simulink library "ESSLibrary"  (R2020a)
settings: Solver=VariableStepAuto  StartTime=0.0  StopTime=10.0  RelTol=1e-3
libraries: $bdroot x82, powerlib_meascontrol x10, simulink x7
(part 1 of 7)
settings Model: Creator=ASHUTOSHKUMARTIWARI  LastModifiedBy=soumyakantapanda

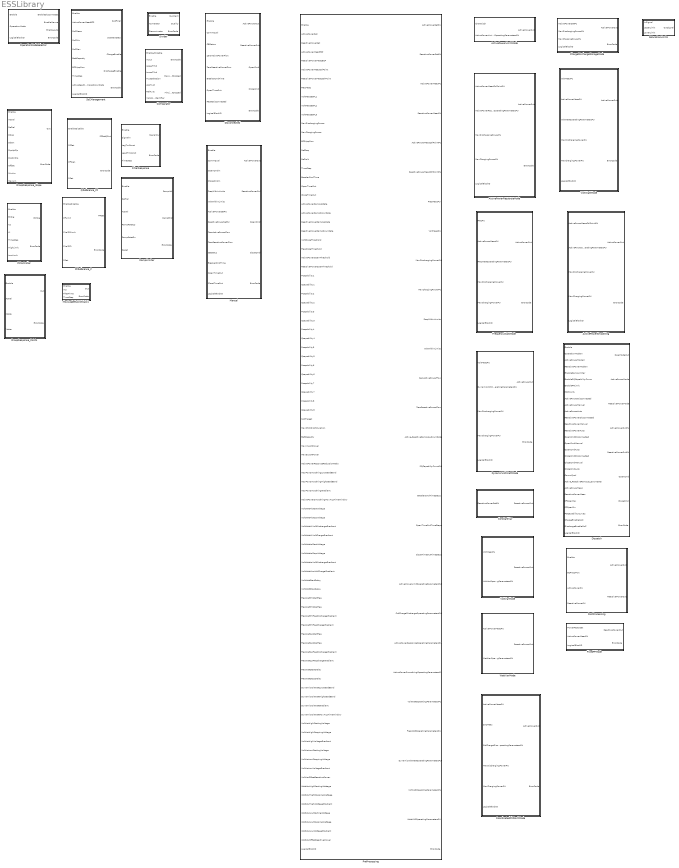
== system ESSLibrary ==
  ActivePowerLimitMode : Subsystem  RTWFcnName=ActivePowerLimitMode
      settings: RTWFcnNameOpts=User specified  RTWFileNameOpts=Use function name
  ActivePowerResponseMode : Subsystem  TreatAsAtomicUnit=on
  ActivePowerSmoothing : Subsystem
  ChargeDischargeStorageMode : Subsystem
  Comparator : Subsystem
  ConstantVar : Subsystem
  CoordinatedChDischMode : Subsystem
  Disconnected : Subsystem  TreatAsAtomicUnit=on  RTWFcnName=Disconnected
      settings: RTWFcnNameOpts=User specified  RTWFileNameOpts=Use function name
  Dispatch : Subsystem
  Divider : Subsystem  TreatAsAtomicUnit=on  RTWFcnName=Divider
      settings: RTWFcnNameOpts=User specified  RTWFileNameOpts=Use function name
  DroopResponse_Points : Subsystem  TreatAsAtomicUnit=on
  DroopResponse_Slope : Subsystem  TreatAsAtomicUnit=on
  DynamicVoltWattMode : Subsystem
  FilterResponse : Subsystem
  FixedPFMode : Subsystem
  FrequencyWattMode : Subsystem  TreatAsAtomicUnit=on
  Manual : Subsystem  TreatAsAtomicUnit=on  RTWFcnName=Manual
      settings: RTWFcnNameOpts=User specified  RTWFileNameOpts=Use function name
  MovAvgDeltaVoltCalc1 : Subsystem
  OperationModeSelector : Subsystem  TreatAsAtomicUnit=on  RTWFcnName=OperationModeSelector
      settings: RTWFcnNameOpts=User specified  RTWFileNameOpts=Use function name
  PFReference_P : Subsystem  TreatAsAtomicUnit=on
  PIController : Subsystem  TreatAsAtomicUnit=on
  PostProcessing : Subsystem
  PreProcessing : Subsystem  TreatAsAtomicUnit=on  RTWFcnName=PreProcessing
      settings: RTWFcnNameOpts=User specified  RTWFileNameOpts=Use function name
  QReference_PF : Subsystem  TreatAsAtomicUnit=on
  RampLimiter : MATLAB Function  TreatAsAtomicUnit=on
  SaturationLimits : Subsystem
  SoCManagement : Subsystem  TreatAsAtomicUnit=on  RTWFcnName=SoCManagement
      settings: RTWFcnNameOpts=User specified  RTWFileNameOpts=Use function name
  VoltVarMode : Subsystem
  VoltWattMode : Subsystem
  WattVarMode : Subsystem

== system ESSLibrary/ActivePowerLimitMode ==
  ChOrDisch : Inport  OutDataTypeStr=double
  ActivePowerLimitOperatingParametersPU : Inport  Port=2  OutDataTypeStr=Bus: ActivePowerLimitOperatingParametersPU
  Action Port : ActionPort
  Bus Selector1 : BusSelector  OutputSignals=MaxDischargingPowerPU,MaxChargingPowerPU
  Switch : Switch  Criteria=u2 > Threshold
  ActivePowerOut : Outport
  wires:
  ChOrDisch/1 -> Switch/2
  Switch/1 -> ActivePowerOut/1
  ActivePowerLimitOperatingParametersPU/1 -> Bus Selector1/1
  Bus Selector1/1 -> Switch/1  "<MaxDischargingPowerPU>"
  Bus Selector1/2 -> Switch/3  "<MaxChargingPowerPU>"

== system ESSLibrary/ActivePowerResponseMode ==
  ActivePowerMeasCtrlPointPU : Inport  OutDataTypeStr=double
  ActivePowerResponseOperatingParametersPU : Inport  Port=2  OutDataTypeStr=Bus: ActivePowerResponseOperatingParametersPU
  MaxDischargingPowerPU : Inport  Port=3  OutDataTypeStr=double
  MaxChargingPowerPU : Inport  Port=4  OutDataTypeStr=double
  LogicalBlockID : Inport  Port=5  OutDataTypeStr=int64
  Action Port : ActionPort
  ActivePowerMeasCtrlPointPU1 : InportShadow  OutDataTypeStr=double
  Bus Selector6 : BusSelector  OutputSignals=MaxExportPowerPU,MaxImportPowerPU,ReductionRatio
  Comparator : $bdroot/ChargeDischargeStorageMode/Comparator  SystemSampleTime=-1  Latency=0  AutoFrameSizeCalculation=off
  Constant10 : Constant  Value=0  OutDataTypeStr=int64
  Constant11 : Constant  Value=0  OutDataTypeStr=int64
  Constant2 : Constant  Value=2  OutDataTypeStr=int32
  Constant3 : Constant  Value=0  OutDataTypeStr=int8
  Constant5 : Constant  Value=0  OutDataTypeStr=int8
  Constant6 : Constant  OutDataTypeStr=boolean
  Divide1 : Product  Inputs=**
  Divide2 : Product  Inputs=**
  Equal2 : RelationalOperator  Operator=>  OutDataTypeStr=boolean  RndMeth=Simplest
  Gain1 : Gain  Gain=1000000
  Less Than : RelationalOperator  OutDataTypeStr=boolean  RndMeth=Simplest
  Less Than1 : RelationalOperator  Operator=<=  OutDataTypeStr=boolean  RndMeth=Simplest
  MaxChargingPowerPU1 : InportShadow  Port=4  OutDataTypeStr=double
  MaxDischargingPowerPU1 : InportShadow  Port=3  OutDataTypeStr=double
  SaturationLimits : $bdroot/SaturationLimits  SystemSampleTime=-1  Latency=0  AutoFrameSizeCalculation=off
  Sum : Sum  Inputs=|+-
  Sum1 : Sum  Inputs=|-+
  Sum2 : Sum  OutDataTypeStr=int64
  Switch : Switch  Criteria=u2 > Threshold  OutDataTypeStr=double
  Switch1 : Switch  Criteria=u2 > Threshold  OutDataTypeStr=double
  Switch4 : Switch  Criteria=u2 > Threshold
  Terminator : Terminator
  Terminator1 : Terminator
  VariableIdentifier : Constant  OutDataTypeStr=int64
  Zero : Constant  Value=0.0  OutDataTypeStr=double
  ActivePowerOut : Outport
  ErrorCode : Outport  Port=2  OutDataTypeStr=int64
  wires:
  [ReductionRatio] -> Divide1/2
  Divide1/1 -> Switch/1
  Less Than/1 -> Switch/2
  Sum/1 -> Divide1/1
  ActivePowerResponseOperatingParametersPU/1 -> Bus Selector6/1
  Bus Selector6/1 -> [MaxExportPowerPU]  "<MaxExportPowerPU>"
  Bus Selector6/2 -> [MaxImportPowerPU]  "<MaxImportPowerPU>"
  ActivePowerMeasCtrlPointPU/1 -> Sum/1, Less Than/1
  [MaxExportPowerPU] -> Less Than/2, Sum/2
  Bus Selector6/3 -> [ReductionRatio]  "<ReductionRatio>"
  [MaxImportPowerPU] -> Sum1/2, Less Than1/2
  ActivePowerMeasCtrlPointPU1/1 -> Sum1/1, Less Than1/1
  Less Than1/1 -> Switch1/2
  Switch1/1 -> Switch/3
  Sum1/1 -> Divide2/1
  [ReductionRatio] -> Divide2/2
  Divide2/1 -> Switch1/1
  Zero/1 -> Switch1/3
  Switch/1 -> SaturationLimits/1, Comparator/2
  SaturationLimits/1 -> ActivePowerOut/1
  MaxDischargingPowerPU/1 -> SaturationLimits/2
  MaxChargingPowerPU/1 -> SaturationLimits/3
  Constant10/1 -> Equal2/2
  Sum2/1 -> Switch4/1
  Constant3/1 -> Comparator/6
  Gain1/1 -> Sum2/2
  Equal2/1 -> Switch4/2
  Comparator/1 -> Equal2/1, Sum2/1
  Switch4/1 -> ErrorCode/1
  Constant6/1 -> Comparator/1
  Comparator/2 -> Terminator/1
  Constant11/1 -> Switch4/3
  VariableIdentifier/1 -> Comparator/8
  LogicalBlockID/1 -> Gain1/1
  Constant5/1 -> Comparator/7
  Constant2/1 -> Comparator/5
  Comparator/3 -> Terminator1/1
  MaxDischargingPowerPU1/1 -> Comparator/3
  MaxChargingPowerPU1/1 -> Comparator/4

== system ESSLibrary/ActivePowerSmoothing ==
  ActivePowerMeasCtrlPointPU : Inport
  ActivePowerSmoothingOperatingParametersPU : Inport  Port=2  OutDataTypeStr=Bus: ActivePowerSmoothingParametersPU
  MaxDischargingPowerPU : Inport  Port=3  OutDataTypeStr=double
  MaxChargingPowerPU : Inport  Port=4  OutDataTypeStr=double
  LogicalBlockID : Inport  Port=5  OutDataTypeStr=int64
  Action Port : ActionPort
  ActivePowerMeasCtrlPointPU1 : InportShadow
  Bus Selector2 : BusSelector  OutputSignals=ActivePowerSmoothingLowDeadBandPU,ActivePowerSmoothingHighDeadBandPU,ActivePowerSmoothingGradientPU,ActivePowerSmoothingMovAvgTimeWindow,TimeStep
  Comparator : $bdroot/ChargeDischargeStorageMode/Comparator  SystemSampleTime=-1  Latency=0  AutoFrameSizeCalculation=off
  Constant1 : Constant  Value=0.0  OutDataTypeStr=double  SampleTime=-1
  Constant10 : Constant  Value=0  OutDataTypeStr=int64
  Constant11 : Constant  Value=0  OutDataTypeStr=int64
  Constant2 : Constant  Value=0.0  OutDataTypeStr=double  SampleTime=-1
  Constant3 : Constant  OutDataTypeStr=boolean
  Constant4 : Constant  Value=2  OutDataTypeStr=int32
  Constant5 : Constant  Value=0  OutDataTypeStr=int8
  Constant6 : Constant  Value=0  OutDataTypeStr=int8
  Constant7 : Constant  OutDataTypeStr=boolean
  Equal2 : RelationalOperator  Operator=>  OutDataTypeStr=boolean  RndMeth=Simplest
  Gain1 : Gain  Gain=1000000
  MATLAB Function : MATLAB Function  TreatAsAtomicUnit=on
  MaxChargingPowerPU1 : InportShadow  Port=4  OutDataTypeStr=double
  MaxDischargingPowerPU1 : InportShadow  Port=3  OutDataTypeStr=double
  MovAvgDeltaVoltCalc : Subsystem
  Mux : Mux  Inputs=2
  SaturationLimits : $bdroot/SaturationLimits  SystemSampleTime=-1  Latency=0  AutoFrameSizeCalculation=off
  Sum2 : Sum  OutDataTypeStr=int64
  Switch4 : Switch  Criteria=u2 > Threshold
  Terminator : Terminator
  Terminator1 : Terminator
  VariableIdentifier : Constant  OutDataTypeStr=int64
  ActivePowerOut : Outport
  ErrorCode : Outport  Port=2  OutDataTypeStr=int64
  wires:
  ActivePowerSmoothingOperatingParametersPU/1 -> Bus Selector2/1
  MovAvgDeltaVoltCalc/1(Out) -> MATLAB Function/1(X_In)
  Constant3/1 -> MovAvgDeltaVoltCalc/1(Enable)
  Constant2/1 -> MATLAB Function/3(Y_Offset)
  [TimeStep] -> MovAvgDeltaVoltCalc/4(TimeStep)
  [ActivePowerSmoothingMovAvgTimeWindow] -> MovAvgDeltaVoltCalc/3(FilterTime)
  ActivePowerMeasCtrlPointPU/1 -> MovAvgDeltaVoltCalc/2(Inp)
  Bus Selector2/1 -> [ActivePowerSmoothingLowDeadBandPU]  "<ActivePowerSmoothingLowDeadBandPU>"
  Bus Selector2/2 -> [ActivePowerSmoothingHighDeadBandPU]  "<ActivePowerSmoothingHighDeadBandPU>"
  Bus Selector2/3 -> [ActivePowerSmoothingGradientPU]  "<ActivePowerSmoothingGradientPU>"
  Bus Selector2/4 -> [ActivePowerSmoothingMovAvgTimeWindow]  "<ActivePowerSmoothingMovAvgTimeWindow>"
  ActivePowerMeasCtrlPointPU1/1 -> MATLAB Function/2(X_Ref)
  Bus Selector2/5 -> [TimeStep]  "<TimeStep>"
  [ActivePowerSmoothingHighDeadBandPU] -> MATLAB Function/4(X_Hi_Deadband)
  [ActivePowerSmoothingLowDeadBandPU] -> MATLAB Function/5(X_Lo_Deadband)
  [ActivePowerSmoothingGradientPU] -> MATLAB Function/7(X_Lo_Gradient), MATLAB Function/6(X_Hi_Gradient)
  Constant1/1 -> MATLAB Function/9(StopDelay), MATLAB Function/8(StartDelay)
  SaturationLimits/1 -> ActivePowerOut/1
  MaxChargingPowerPU/1 -> SaturationLimits/3
  MaxDischargingPowerPU/1 -> SaturationLimits/2
  Constant11/1 -> Switch4/3
  Gain1/1 -> Sum2/2
  Equal2/1 -> Switch4/2
  MaxDischargingPowerPU1/1 -> Comparator/3
  Comparator/3 -> Terminator1/1
  Sum2/1 -> Switch4/1
  MATLAB Function/1(Y_Out) -> Comparator/2, SaturationLimits/1
  MaxChargingPowerPU1/1 -> Comparator/4
  Constant10/1 -> Equal2/2
  LogicalBlockID/1 -> Gain1/1
  Constant6/1 -> Comparator/7
  Constant4/1 -> Comparator/5
  VariableIdentifier/1 -> Comparator/8
  Constant7/1 -> Comparator/1
  Comparator/1 -> Equal2/1, Sum2/1
  Constant5/1 -> Comparator/6
  Comparator/2 -> Terminator/1
  MovAvgDeltaVoltCalc/2(ErrorCode) -> [MovAvgErrorCode]
  Switch4/1 -> Mux/1
  [MovAvgErrorCode] -> Mux/2
  Mux/1 -> ErrorCode/1

== system ESSLibrary/ChargeDischargeStorageMode ==
  ActivePowerSetPU : Inport  OutDataTypeStr=double
  MaxDischargingPowerPU : Inport  Port=2  OutDataTypeStr=double
  MaxChargingPowerPU : Inport  Port=3  OutDataTypeStr=double
  LogicalBlockID : Inport  Port=4  OutDataTypeStr=int64
  Action Port : ActionPort
  ActivePowerSetPU1 : InportShadow  OutDataTypeStr=double
  Comparator : Subsystem
  Constant10 : Constant  Value=0  OutDataTypeStr=int64
  Constant11 : Constant  Value=0  OutDataTypeStr=int64
  Constant2 : Constant  Value=2  OutDataTypeStr=int32
  Constant3 : Constant  Value=0  OutDataTypeStr=int8
  Constant5 : Constant  Value=0  OutDataTypeStr=int8
  Constant6 : Constant  OutDataTypeStr=boolean
  Equal2 : RelationalOperator  Operator=>  OutDataTypeStr=boolean  RndMeth=Simplest
  GT : RelationalOperator  Operator=>  OutDataTypeStr=boolean  RndMeth=Simplest
  Gain1 : Gain  Gain=1000000
  LT : RelationalOperator  Operator=<  OutDataTypeStr=boolean  RndMeth=Simplest
  MaxChargingPowerPU1 : InportShadow  Port=3  OutDataTypeStr=double
  MaxDischargingPowerPU1 : InportShadow  Port=2  OutDataTypeStr=double
  Sum1 : Sum  OutDataTypeStr=int64
  Switch : Switch  Criteria=u2 > Threshold
  Switch1 : Switch  Criteria=u2 > Threshold
  Switch4 : Switch  Criteria=u2 > Threshold
  Terminator : Terminator
  Terminator1 : Terminator
  VariableIdentifier : Constant  OutDataTypeStr=int64
  ActivePowerOut : Outport
  ErrorCode : Outport  Port=2  OutDataTypeStr=int64
  wires:
  ActivePowerSetPU/1 -> Switch/1, GT/1
  MaxDischargingPowerPU/1 -> Switch/3, GT/2
  GT/1 -> Switch/2
  Switch/1 -> Switch1/1, LT/1
  MaxChargingPowerPU/1 -> Switch1/3, LT/2
  LT/1 -> Switch1/2
  Switch1/1 -> ActivePowerOut/1
  Constant6/1 -> Comparator/1(Enable/Disable)
  Constant5/1 -> Comparator/7(RelHyst)
  VariableIdentifier/1 -> Comparator/8(VariableIdentifier)
  MaxDischargingPowerPU1/1 -> Comparator/3(UpperTrhd)
  Comparator/3(MinLimitCrossed) -> Terminator1/1
  Comparator/2(MaxLimitCrossed) -> Terminator/1
  LogicalBlockID/1 -> Gain1/1
  Comparator/1(ErrorCode) -> Equal2/1, Sum1/1
  Gain1/1 -> Sum1/2
  Constant3/1 -> Comparator/6(AbsHyst)
  Sum1/1 -> Switch4/1
  MaxChargingPowerPU1/1 -> Comparator/4(LowerTrhd)
  Equal2/1 -> Switch4/2
  Constant11/1 -> Switch4/3
  Constant10/1 -> Equal2/2
  Switch4/1 -> ErrorCode/1
  Constant2/1 -> Comparator/5(HystSelection)
  ActivePowerSetPU1/1 -> Comparator/2("Input ")

== system ESSLibrary/Comparator ==
  note: LowerThresholdID
  note: UpperThresholdID
  note: CategoryID = 1
  Enable/Disable : Inport
  "Input " : Inport  Port=2
  UpperTrhd : Inport  Port=3
  LowerTrhd : Inport  Port=4
  HystSelection : Inport  Port=5
  AbsHyst : Inport  Port=6
  RelHyst : Inport  Port=7
  VariableIdentifier : Inport  Port=8
  Basic alarm ver2.0 : Subsystem
  CategoryID : Constant  OutDataTypeStr=int64
  Constant1 : Constant  OutDataTypeStr=int64
  Constant10 : Constant  Value=0  OutDataTypeStr=int64
  Constant11 : Constant  Value=0  OutDataTypeStr=int64
  Constant2 : Constant  Value=2  OutDataTypeStr=int64
  Gain : Gain  Gain=100
  Gain1 : Gain  Gain=10000
  Sum : Sum  Inputs=+++  OutDataTypeStr=int64
  Switch1 : Switch  Criteria=u2 ~= 0  OutDataTypeStr=int64
  Switch2 : Switch  Criteria=u2 ~= 0  OutDataTypeStr=int64
  Switch3 : Switch  Criteria=u2 ~= 0  OutDataTypeStr=int64
  Terminator1 : Terminator
  ErrorCode : Outport
  MaxLimitCrossed : Outport  Port=2
  MinLimitCrossed : Outport  Port=3
  wires:
  Basic alarm ver2.0/1(MaxLimitCrossed) -> MaxLimitCrossed/1, Switch1/2
  Constant2/1 -> Switch2/1
  CategoryID/1 -> Gain/1
  Switch1/1 -> Switch3/2, Sum/1
  Constant1/1 -> Switch1/1
  Constant11/1 -> Switch2/3
  HystSelection/1 -> Basic alarm ver2.0/5(HystSelection)
  Basic alarm ver2.0/2(MinLimitCrossed) -> MinLimitCrossed/1, Switch2/2
  Constant10/1 -> Switch3/3
  Basic alarm ver2.0/3(ErrorCode) -> Terminator1/1
  Sum/1 -> Switch3/1
  "Input "/1 -> Basic alarm ver2.0/2("Input ")
  Switch2/1 -> Switch1/3
  VariableIdentifier/1 -> Gain1/1
  AbsHyst/1 -> Basic alarm ver2.0/6(AbsHyst)
  RelHyst/1 -> Basic alarm ver2.0/7(RelHyst)
  Enable/Disable/1 -> Basic alarm ver2.0/1(Enable/disable)
  Switch3/1 -> ErrorCode/1
  UpperTrhd/1 -> Basic alarm ver2.0/3(UpperTrhd)
  LowerTrhd/1 -> Basic alarm ver2.0/4(LowerTrhd)
  Gain/1 -> Sum/2
  Gain1/1 -> Sum/3

== system ESSLibrary/ConstantVar ==
  ReactivePowerSetPU : Inport
  Action Port : ActionPort
  ReactivePowerOut : Outport  OutDataTypeStr=double
  wires:
  ReactivePowerSetPU/1 -> ReactivePowerOut/1

== system ESSLibrary/CoordinatedChDischMode ==
  ActivePowerMeasPU : Inport
  SoCMeas : Inport  Port=2  OutDataTypeStr=double
  CrdChargeDischargeOperatingParametersPU : Inport  Port=3  OutDataTypeStr=Bus: CrdChargeDischargeOperatingParametersPU
  MaxDischargingPowerPU : Inport  Port=4  OutDataTypeStr=double
  MaxChargingPowerPU : Inport  Port=5  OutDataTypeStr=double
  LogicalBlockID : Inport  Port=6  OutDataTypeStr=int64
  Action Port : ActionPort
  Bus Selector : BusSelector  OutputSignals=SoCTarget,MaxChOrDischDuration,BattCapacity,ActivePowerRampUpRatePU,ActivePowerRampDownRatePU,TimeStep,ECPAppPow
  Comparator : $bdroot/ChargeDischargeStorageMode/Comparator  SystemSampleTime=-1  Latency=0  AutoFrameSizeCalculation=off
  Constant10 : Constant  Value=0  OutDataTypeStr=int64
  Constant11 : Constant  Value=0  OutDataTypeStr=int64
  Constant4 : Constant  Value=2  OutDataTypeStr=int32
  Constant5 : Constant  Value=0  OutDataTypeStr=int8
  Constant6 : Constant  Value=0  OutDataTypeStr=int8
  Constant7 : Constant  OutDataTypeStr=boolean
  Divide1 : Product  Inputs=**
  Divide2 : Product  Inputs=**
  Divide3 : Product  Inputs=*/
  Divide4 : Product  Inputs=**
  EnabledCoordinatedChDischMode : Subsystem
  Equal2 : RelationalOperator  Operator=>  OutDataTypeStr=boolean  RndMeth=Simplest
  Gain2 : Gain  Gain=1000000
  MaxChargingPowerPU1 : InportShadow  Port=5  OutDataTypeStr=double
  MaxDischargingPowerPU1 : InportShadow  Port=4  OutDataTypeStr=double
  Mux : Mux  Inputs=2
  SaturationLimits : $bdroot/SaturationLimits  SystemSampleTime=-1  Latency=0  AutoFrameSizeCalculation=off
  Sum2 : Sum  OutDataTypeStr=int64
  Switch4 : Switch  Criteria=u2 > Threshold
  Terminator1 : Terminator
  Terminator2 : Terminator
  VariableIdentifier : Constant  OutDataTypeStr=int64
  ActivePowerOut : Outport
  ErrorCode : Outport  Port=2
  wires:
  SoCMeas/1 -> EnabledCoordinatedChDischMode/2(SoC)
  [BattCapacity] -> EnabledCoordinatedChDischMode/4(BattCapacity)
  [SocTarget] -> EnabledCoordinatedChDischMode/5(TargetSOC)
  [MaxChOrDischDuration] -> EnabledCoordinatedChDischMode/6(MinChargeDuration)
  [ECPAppPow] -> Divide4/1
  [ECPAppPow] -> Divide1/1
  Divide1/1 -> EnabledCoordinatedChDischMode/8(ActivePowerRampDownRate)
  Divide4/1 -> EnabledCoordinatedChDischMode/7(ActivePowerRampUpRate)
  Divide2/1 -> EnabledCoordinatedChDischMode/1(ActvPowMeasPU)
  [ECPAppPow] -> Divide3/2
  EnabledCoordinatedChDischMode/1(ActivePowerOut) -> Divide3/1
  CrdChargeDischargeOperatingParametersPU/1 -> Bus Selector/1
  ActivePowerMeasPU/1 -> Divide2/1
  Bus Selector/7 -> [ECPAppPow]  "<ECPAppPow>"
  [ECPAppPow] -> Divide2/2
  Bus Selector/1 -> [SocTarget]  "<SoCTarget>"
  Bus Selector/2 -> [MaxChOrDischDuration]  "<MaxChOrDischDuration>"
  Bus Selector/3 -> [BattCapacity]  "<BattCapacity>"
  Bus Selector/4 -> [ActivePowerRampUpRatePU]  "<ActivePowerRampUpRatePU>"
  Bus Selector/5 -> [ActivePowerRampDownRatePU]  "<ActivePowerRampDownRatePU>"
  [ActivePowerRampUpRatePU] -> Divide4/2
  [ActivePowerRampDownRatePU] -> Divide1/2
  Bus Selector/6 -> [TimeStep]  "<TimeStep>"
  [TimeStep] -> EnabledCoordinatedChDischMode/3(TimeStep)
  Constant5/1 -> Comparator/6
  Divide3/1 -> SaturationLimits/1, Comparator/2
  [FailOperationErrorCode] -> Mux/1
  Mux/1 -> Sum2/1, Equal2/1
  Constant10/1 -> Equal2/2
  VariableIdentifier/1 -> Comparator/8
  Constant11/1 -> Switch4/3
  MaxChargingPowerPU1/1 -> Comparator/4
  Switch4/1 -> ErrorCode/1
  Gain2/1 -> Sum2/2
  Comparator/1 -> Mux/2
  MaxDischargingPowerPU1/1 -> Comparator/3
  Constant4/1 -> Comparator/5
  MaxDischargingPowerPU/1 -> SaturationLimits/2
  Comparator/3 -> Terminator2/1
  MaxChargingPowerPU/1 -> SaturationLimits/3
  Constant7/1 -> Comparator/1
  Equal2/1 -> Switch4/2
  SaturationLimits/1 -> ActivePowerOut/1
  LogicalBlockID/1 -> Gain2/1
  Sum2/1 -> Switch4/1
  Constant6/1 -> Comparator/7
  Comparator/2 -> Terminator1/1
  EnabledCoordinatedChDischMode/2(FailOperationErrorCode) -> [FailOperationErrorCode]

== system ESSLibrary/Disconnected ==
  Enable : Inport  OutDataTypeStr=boolean
  CommQual : Inport  Port=2  OutDataTypeStr=boolean
  CBStatus : Inport  Port=3  OutDataTypeStr=int8
  ZeroActivePowerFlow : Inport  Port=4  OutDataTypeStr=boolean
  ZeroReactivePowerFlow : Inport  Port=5  OutDataTypeStr=boolean
  BreakerCmdTime : Inport  Port=6
  OpenTimeOut : Inport  Port=7
  ResetDisconnected : Inport  Port=8
  LogicalBlockID : Inport  Port=9  OutDataTypeStr=int64
  AND : Logic  IconShape=distinctive  AllPortsSameDT=off  OutDataTypeStr=boolean
  If : If  IfExpression=u1 ~= 0
  If Action Subsystem : Subsystem  TreatAsAtomicUnit=on
  IfActionSubsystem : Subsystem  TreatAsAtomicUnit=on
  NOT : Logic  Operator=NOT  IconShape=distinctive  AllPortsSameDT=off  OutDataTypeStr=boolean
  Switch{,1..4} (5 alike) : Switch  Criteria=u2 > Threshold
  ActivePowerOut : Outport
  ReactivePowerOut : Outport  Port=2
  OpenCmd : Outport  Port=3
  CloseCmd : Outport  Port=4
  ErrorCode : Outport  Port=5  OutDataTypeStr=int64
  wires:
  If/1 -> IfActionSubsystem/Action
  If/2 -> If Action Subsystem/Action
  If Action Subsystem/3(OpenCmd) -> [ElseOpenCmd]
  If Action Subsystem/4(CloseCmd) -> [ElseCloseCmd]
  If Action Subsystem/1(ActivePowerOut) -> [ElseActivePowerOut]
  If Action Subsystem/2(ReactivePowerOut) -> [ElseReactivePowerOut]
  If Action Subsystem/5(ErrorCode) -> [ElseErrorCode]
  IfActionSubsystem/2(ReactivePowerOut) -> [IfReactivePowerOut]
  IfActionSubsystem/1(ActivePowerOut) -> [IfActivePowerOut]
  IfActionSubsystem/3(OpenCmd) -> [IfOpenCmd]
  IfActionSubsystem/4(CloseCmd) -> [IfCloseCmd]
  IfActionSubsystem/5(ErrorCode) -> [IfErrorCode]
  CommQual/1 -> NOT/1
  Enable/1 -> AND/1
  AND/1 -> Switch/2, Switch1/2, Switch2/2, Switch3/2, Switch4/2, If/1
  NOT/1 -> AND/2
  CBStatus/1 -> IfActionSubsystem/1(CBStatus)
  ZeroActivePowerFlow/1 -> IfActionSubsystem/2(ZeroActivePowerFlow)
  ZeroReactivePowerFlow/1 -> IfActionSubsystem/3(ZeroReactivePowerFlow)
  BreakerCmdTime/1 -> IfActionSubsystem/4(BreakerCmdTime)
  [IfActivePowerOut] -> Switch/1
  [ElseActivePowerOut] -> Switch/3
  [IfReactivePowerOut] -> Switch1/1
  [ElseReactivePowerOut] -> Switch1/3
  [IfOpenCmd] -> Switch2/1
  [ElseOpenCmd] -> Switch2/3
  [IfCloseCmd] -> Switch3/1
  [ElseCloseCmd] -> Switch3/3
  [IfErrorCode] -> Switch4/1
  [ElseErrorCode] -> Switch4/3
  LogicalBlockID/1 -> IfActionSubsystem/7(LogicalBlockID)
  Switch/1 -> ActivePowerOut/1
  Switch1/1 -> ReactivePowerOut/1
  Switch2/1 -> OpenCmd/1
  Switch3/1 -> CloseCmd/1
  Switch4/1 -> ErrorCode/1
  OpenTimeOut/1 -> IfActionSubsystem/5(OpenTimeOut)
  ResetDisconnected/1 -> IfActionSubsystem/6(ResetDisconnected)

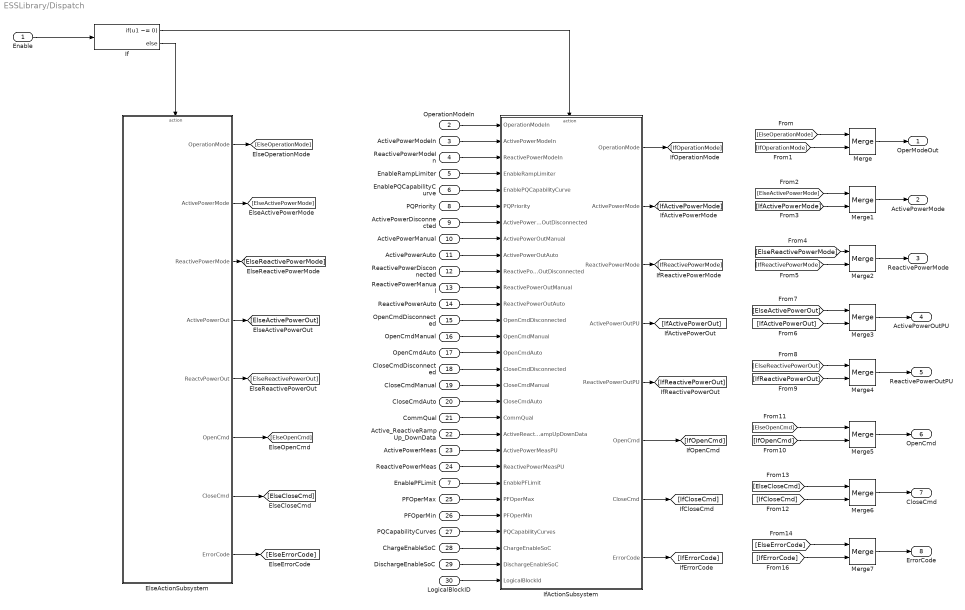
== system ESSLibrary/Dispatch ==
  Enable : Inport
  OperationModeIn : Inport  Port=2
  ActivePowerModeIn : Inport  Port=3
  ReactivePowerModeIn : Inport  Port=4
  EnableRampLimiter : Inport  Port=5
  EnablePQCapabilityCurve : Inport  Port=6
  EnablePFLimit : Inport  Port=7
  PQPriority : Inport  Port=8
  ActivePowerDisconnected : Inport  Port=9
  ActivePowerManual : Inport  Port=10
  ActivePowerAuto : Inport  Port=11
  ReactivePowerDisconnected : Inport  Port=12
  ReactivePowerManual : Inport  Port=13
  ReactivePowerAuto : Inport  Port=14
  OpenCmdDisconnected : Inport  Port=15
  OpenCmdManual : Inport  Port=16
  OpenCmdAuto : Inport  Port=17
  CloseCmdDisconnected : Inport  Port=18
  CloseCmdManual : Inport  Port=19
  CloseCmdAuto : Inport  Port=20
  CommQual : Inport  Port=21
  Active_ReactiveRampUp_DownData : Inport  Port=22
  ActivePowerMeas : Inport  Port=23
  ReactivePowerMeas : Inport  Port=24
  PFOperMax : Inport  Port=25
  PFOperMin : Inport  Port=26
  PQCapabilityCurves : Inport  Port=27
  ChargeEnableSoC : Inport  Port=28
  DischargeEnableSoC : Inport  Port=29
  LogicalBlockID : Inport  Port=30
  ElseActionSubsystem : Subsystem  TreatAsAtomicUnit=on
  If : If  IfExpression=u1 ~= 0
  IfActionSubsystem : Subsystem  TreatAsAtomicUnit=on
  Merge{,1..7} (8 alike) : Merge
  OperModeOut : Outport
  ActivePowerMode : Outport  Port=2
  ReactivePowerMode : Outport  Port=3
  ActivePowerOutPU : Outport  Port=4
  ReactivePowerOutPU : Outport  Port=5
  OpenCmd : Outport  Port=6
  CloseCmd : Outport  Port=7
  ErrorCode : Outport  Port=8
  wires:
  ElseActionSubsystem/7(CloseCmd) -> [ElseCloseCmd]
  ElseActionSubsystem/4(ActivePowerOut) -> [ElseActivePowerOut]
  ElseActionSubsystem/6(OpenCmd) -> [ElseOpenCmd]
  Enable/1 -> If/1
  Merge2/1 -> ReactivePowerMode/1
  Merge/1 -> OperModeOut/1
  If/2 -> ElseActionSubsystem/Action
  If/1 -> IfActionSubsystem/Action
  Merge6/1 -> CloseCmd/1
  ElseActionSubsystem/5(ReactvPowerOut) -> [ElseReactivePowerOut]
  ElseActionSubsystem/1(OperationMode) -> [ElseOperationMode]
  Merge1/1 -> ActivePowerMode/1
  Merge5/1 -> OpenCmd/1
  Merge4/1 -> ReactivePowerOutPU/1
  Merge3/1 -> ActivePowerOutPU/1
  ElseActionSubsystem/8(ErrorCode) -> [ElseErrorCode]
  Merge7/1 -> ErrorCode/1
  ElseActionSubsystem/2(ActivePowerMode) -> [ElseActivePowerMode]
  ElseActionSubsystem/3(ReactivePowerMode) -> [ElseReactivePowerMode]
  OperationModeIn/1 -> IfActionSubsystem/1(OperationModeIn)
  ActivePowerModeIn/1 -> IfActionSubsystem/2(ActivePowerModeIn)
  ReactivePowerModeIn/1 -> IfActionSubsystem/3(ReactivePowerModeIn)
  EnablePQCapabilityCurve/1 -> IfActionSubsystem/5(EnablePQCapabilityCurve)
  ActivePowerDisconnected/1 -> IfActionSubsystem/7(ActivePowerOutDisconnected)
  ActivePowerManual/1 -> IfActionSubsystem/8(ActivePowerOutManual)
  ActivePowerAuto/1 -> IfActionSubsystem/9(ActivePowerOutAuto)
  ReactivePowerDisconnected/1 -> IfActionSubsystem/10(ReactivePowerOutDisconnected)
  ReactivePowerManual/1 -> IfActionSubsystem/11(ReactivePowerOutManual)
  PQPriority/1 -> IfActionSubsystem/6(PQPriority)
  ReactivePowerAuto/1 -> IfActionSubsystem/12(ReactivePowerOutAuto)
  OpenCmdDisconnected/1 -> IfActionSubsystem/13(OpenCmdDisconnected)
  OpenCmdManual/1 -> IfActionSubsystem/14(OpenCmdManual)
  OpenCmdAuto/1 -> IfActionSubsystem/15(OpenCmdAuto)
  CloseCmdDisconnected/1 -> IfActionSubsystem/16(CloseCmdDisconnected)
  CloseCmdManual/1 -> IfActionSubsystem/17(CloseCmdManual)
  CloseCmdAuto/1 -> IfActionSubsystem/18(CloseCmdAuto)
  CommQual/1 -> IfActionSubsystem/19(CommQual)
  Active_ReactiveRampUp_DownData/1 -> IfActionSubsystem/20(ActiveReactiveRampUpDownData)
  ActivePowerMeas/1 -> IfActionSubsystem/21(ActivePowerMeasPU)
  ReactivePowerMeas/1 -> IfActionSubsystem/22(ReactivePowerMeasPU)
  EnablePFLimit/1 -> IfActionSubsystem/23(EnablePFLimit)
  PFOperMax/1 -> IfActionSubsystem/24(PFOperMax)
  PFOperMin/1 -> IfActionSubsystem/25(PFOperMin)
  PQCapabilityCurves/1 -> IfActionSubsystem/26(PQCapabilityCurves)
  DischargeEnableSoC/1 -> IfActionSubsystem/28(DischargeEnableSoC)
  ChargeEnableSoC/1 -> IfActionSubsystem/27(ChargeEnableSoC)
  EnableRampLimiter/1 -> IfActionSubsystem/4(EnableRampLimiter)
  IfActionSubsystem/1(OperationMode) -> [IfOperationMode]
  IfActionSubsystem/2(ActivePowerMode) -> [IfActivePowerMode]
  IfActionSubsystem/3(ReactivePowerMode) -> [IfReactivePowerMode]
  IfActionSubsystem/8(ErrorCode) -> [IfErrorCode]
  IfActionSubsystem/4(ActivePowerOutPU) -> [IfActivePowerOut]
  IfActionSubsystem/5(ReactivePowerOutPU) -> [IfReactivePowerOut]
  IfActionSubsystem/7(CloseCmd) -> [IfCloseCmd]
  IfActionSubsystem/6(OpenCmd) -> [IfOpenCmd]
  [ElseOperationMode] -> Merge/1
  [IfOperationMode] -> Merge/2
  [ElseActivePowerMode] -> Merge1/1
  [IfActivePowerMode] -> Merge1/2
  [ElseReactivePowerMode] -> Merge2/1
  [IfReactivePowerMode] -> Merge2/2
  [ElseActivePowerOut] -> Merge3/1
  [IfActivePowerOut] -> Merge3/2
  [IfReactivePowerOut] -> Merge4/2
  [ElseReactivePowerOut] -> Merge4/1
  [IfOpenCmd] -> Merge5/2
  [ElseOpenCmd] -> Merge5/1
  [IfCloseCmd] -> Merge6/2
  [ElseCloseCmd] -> Merge6/1
  [IfErrorCode] -> Merge7/2
  [ElseErrorCode] -> Merge7/1
  LogicalBlockID/1 -> IfActionSubsystem/29(LogicalBlockId)

== system ESSLibrary/Divider ==
  Enable : Inport  OutDataTypeStr=boolean
  Numerator : Inport  Port=2
  Denominator : Inport  Port=3
  ElseActionSubsystem : Subsystem  TreatAsAtomicUnit=on
  If : If  IfExpression=u1 ~= 0
  IfActionSubsystem : Subsystem  TreatAsAtomicUnit=on
  Switch6 : Switch  Criteria=u2 > Threshold
  Switch7 : Switch  Criteria=u2 > Threshold
  Switch8 : Switch  Criteria=u2 > Threshold
  Quotient : Outport
  Quality : Outport  Port=2  OutDataTypeStr=boolean
  ErrorCode : Outport  Port=3  OutDataTypeStr=int64
  wires:
  Enable/1 -> If/1, Switch6/2, Switch7/2, Switch8/2
  Numerator/1 -> IfActionSubsystem/1(Numerator)
  [ElseQuotient] -> Switch7/3
  IfActionSubsystem/1(Quality) -> [IfQuality]
  If/2 -> ElseActionSubsystem/Action
  ElseActionSubsystem/1(Quality) -> [ElseQuality]
  Switch6/1 -> Quality/1
  Denominator/1 -> IfActionSubsystem/2(Denominator)
  Switch7/1 -> Quotient/1
  [ElseQuality] -> Switch6/3
  IfActionSubsystem/3(ErrorCode) -> [IfErrorCode]
  IfActionSubsystem/2(Out) -> [IfQuotient]
  ElseActionSubsystem/2(Out) -> [ElseQuotient]
  If/1 -> IfActionSubsystem/Action
  ElseActionSubsystem/3(ErrorCode) -> [ElseErrorCode]
  [IfErrorCode] -> Switch8/1
  [ElseErrorCode] -> Switch8/3
  [IfQuotient] -> Switch7/1
  [IfQuality] -> Switch6/1
  Switch8/1 -> ErrorCode/1

== system ESSLibrary/DroopResponse_Points ==
  Enable : Inport
  ActVal : Inport  Port=2
  Xdata : Inport  Port=3
  Ydata : Inport  Port=4
  Enable1 : InportShadow
  If : If  IfExpression=u1 ~= 0
  If Action Subsystem : Subsystem  TreatAsAtomicUnit=on
  If Action Subsystem2 : Subsystem  TreatAsAtomicUnit=on
  Switch : Switch  Criteria=u2 > Threshold
  Switch1 : Switch  Criteria=u2 > Threshold
  Out : Outport
  ErrorCode : Outport  Port=2
  wires:
  Enable/1 -> If/1
  If/1 -> If Action Subsystem/Action
  If/2 -> If Action Subsystem2/Action
  ActVal/1 -> If Action Subsystem/1(ActVal)
  Xdata/1 -> If Action Subsystem/2(Xdata)
  Ydata/1 -> If Action Subsystem/3(Ydata)
  Switch/1 -> ErrorCode/1
  Switch1/1 -> Out/1
  Enable1/1 -> Switch1/2, Switch/2
  If Action Subsystem/2(ErrorCode) -> [IfErrorCode]
  If Action Subsystem/1(Interpol) -> [IfResOut]
  [ElseErrorCode] -> Switch/3
  [IfErrorCode] -> Switch/1
  [IfResOut] -> Switch1/1
  [ElseResOut] -> Switch1/3
  If Action Subsystem2/2(ErrorCode) -> [ElseErrorCode]
  If Action Subsystem2/1(Out) -> [ElseResOut]

== system ESSLibrary/DroopResponse_Slope ==
  Enable : Inport
  ActVal : Inport  Port=2
  RefVal : Inport  Port=3
  DbUp : Inport  Port=4
  DbDn : Inport  Port=5
  DrpUpSlp : Inport  Port=6
  DrpDnSlp : Inport  Port=7
  Offset : Inport  Port=8
  MinLim : Inport  Port=9
  MaxLim : Inport  Port=10
  Enable1 : InportShadow
  If : If  IfExpression=u1 ~= 0
  If Action Subsystem : Subsystem  TreatAsAtomicUnit=on
  If Action Subsystem1 : Subsystem  TreatAsAtomicUnit=on
  Switch : Switch  Criteria=u2 > Threshold
  Switch1 : Switch  Criteria=u2 > Threshold
  Out : Outport
  ErrorCode : Outport  Port=2
  wires:
  Enable/1 -> If/1
  If/1 -> If Action Subsystem/Action
  If/2 -> If Action Subsystem1/Action
  ActVal/1 -> If Action Subsystem/1(ActVal)
  RefVal/1 -> If Action Subsystem/2(RefVal)
  DbUp/1 -> If Action Subsystem/3(DbUp)
  DbDn/1 -> If Action Subsystem/4(DbDn)
  DrpUpSlp/1 -> If Action Subsystem/5(DrpUpSlp)
  DrpDnSlp/1 -> If Action Subsystem/6(DrpDnSlp)
  Offset/1 -> If Action Subsystem/7(Offset)
  Switch/1 -> ErrorCode/1
  Switch1/1 -> Out/1
  Enable1/1 -> Switch/2, Switch1/2
  If Action Subsystem1/2(ErrorCode) -> [ElseErrorCode]
  If Action Subsystem1/1(ResOut) -> [ElseOut]
  If Action Subsystem/2(ErrorCode) -> [IfErrorCode]
  If Action Subsystem/1(ResOut) -> [IfOut]
  [ElseErrorCode] -> Switch/3
  [IfErrorCode] -> Switch/1
  [IfOut] -> Switch1/1
  [ElseOut] -> Switch1/3
  MaxLim/1 -> If Action Subsystem/9(MaxLim)
  MinLim/1 -> If Action Subsystem/8(MinLim)

== system ESSLibrary/DynamicVoltWattMode ==
  VoltMeasPU : Inport
  DynamicVoltWattOperatingParametersPU : Inport  Port=2  OutDataTypeStr=Bus: DynamicVoltWattOperatingParameters
  MaxDischargingPowerPU : Inport  Port=3  OutDataTypeStr=double
  MaxChargingPowerPU : Inport  Port=4  OutDataTypeStr=double
  LogicalBlockID : Inport  Port=5  OutDataTypeStr=int64
  Action Port : ActionPort
  ActivePowerMeasCtrlPointPU1 : InportShadow
  Bus Selector2 : BusSelector  OutputSignals=DynamicVoltWattLowDeadBandPU,DynamicVoltWattHighDeadBandPU,DynamicVoltWattGradientPU,DynamicVoltWattMovAvgTimeWindow,TimeStep
  Comparator : $bdroot/ChargeDischargeStorageMode/Comparator  SystemSampleTime=-1  Latency=0  AutoFrameSizeCalculation=off
  Constant1 : Constant  Value=0.0  OutDataTypeStr=double  SampleTime=-1
  Constant10 : Constant  Value=0  OutDataTypeStr=int64
  Constant11 : Constant  Value=0  OutDataTypeStr=int64
  Constant2 : Constant  Value=0.0  OutDataTypeStr=double  SampleTime=-1
  Constant3 : Constant  OutDataTypeStr=boolean
  Constant4 : Constant  Value=2  OutDataTypeStr=int32
  Constant5 : Constant  Value=0  OutDataTypeStr=int8
  Constant6 : Constant  Value=0  OutDataTypeStr=int8
  Constant7 : Constant  OutDataTypeStr=boolean
  Equal2 : RelationalOperator  Operator=>  OutDataTypeStr=boolean  RndMeth=Simplest
  Gain1 : Gain  Gain=1000000
  MATLAB Function : MATLAB Function  TreatAsAtomicUnit=on
  MaxChargingPowerPU1 : InportShadow  Port=4  OutDataTypeStr=double
  MaxDischargingPowerPU1 : InportShadow  Port=3  OutDataTypeStr=double
  MovAvgDeltaVoltCalc : Subsystem
  Mux : Mux  Inputs=2
  SaturationLimits : $bdroot/SaturationLimits  SystemSampleTime=-1  Latency=0  AutoFrameSizeCalculation=off
  Sum2 : Sum  OutDataTypeStr=int64
  Switch4 : Switch  Criteria=u2 > Threshold
  Terminator : Terminator
  Terminator1 : Terminator
  VariableIdentifier : Constant  OutDataTypeStr=int64
  ActivePowerOut : Outport
  ErrorCode : Outport  Port=2  OutDataTypeStr=int64
  wires:
  Mux/1 -> ErrorCode/1
  [MovAvgErrorCode] -> Mux/2
  Switch4/1 -> Mux/1
  MovAvgDeltaVoltCalc/2(ErrorCode) -> [MovAvgErrorCode]
  Comparator/2 -> Terminator/1
  Constant5/1 -> Comparator/6
  Comparator/1 -> Sum2/1, Equal2/1
  Constant7/1 -> Comparator/1
  VariableIdentifier/1 -> Comparator/8
  Constant4/1 -> Comparator/5
  Constant6/1 -> Comparator/7
  LogicalBlockID/1 -> Gain1/1
  Constant10/1 -> Equal2/2
  MaxChargingPowerPU1/1 -> Comparator/4
  MATLAB Function/1(Y_Out) -> SaturationLimits/1, Comparator/2
  Sum2/1 -> Switch4/1
  Comparator/3 -> Terminator1/1
  MaxDischargingPowerPU1/1 -> Comparator/3
  Equal2/1 -> Switch4/2
  Gain1/1 -> Sum2/2
  Constant11/1 -> Switch4/3
  MaxDischargingPowerPU/1 -> SaturationLimits/2
  MaxChargingPowerPU/1 -> SaturationLimits/3
  SaturationLimits/1 -> ActivePowerOut/1
  Constant1/1 -> MATLAB Function/8(StartDelay), MATLAB Function/9(StopDelay)
  [DynamicVoltWattGradientPU] -> MATLAB Function/6(X_Hi_Gradient), MATLAB Function/7(X_Lo_Gradient)
  [DynamicVoltWattLowDeadBandPU] -> MATLAB Function/5(X_Lo_Deadband)
  [DynamicVoltWattHighDeadBandPU] -> MATLAB Function/4(X_Hi_Deadband)
  Bus Selector2/5 -> [TimeStep]  "<TimeStep>"
  ActivePowerMeasCtrlPointPU1/1 -> MATLAB Function/2(X_Ref)
  Bus Selector2/4 -> [DynamicVoltWattMovAvgTimeWindow]  "<DynamicVoltWattMovAvgTimeWindow>"
  Bus Selector2/3 -> [DynamicVoltWattGradientPU]  "<DynamicVoltWattGradientPU>"
  Bus Selector2/2 -> [DynamicVoltWattHighDeadBandPU]  "<DynamicVoltWattHighDeadBandPU>"
  Bus Selector2/1 -> [DynamicVoltWattLowDeadBandPU]  "<DynamicVoltWattLowDeadBandPU>"
  VoltMeasPU/1 -> MovAvgDeltaVoltCalc/2(Inp)
  [DynamicVoltWattMovAvgTimeWindow] -> MovAvgDeltaVoltCalc/3(FilterTime)
  [TimeStep] -> MovAvgDeltaVoltCalc/4(TimeStep)
  Constant2/1 -> MATLAB Function/3(Y_Offset)
  Constant3/1 -> MovAvgDeltaVoltCalc/1(Enable)
  MovAvgDeltaVoltCalc/1(Out) -> MATLAB Function/1(X_In)
  DynamicVoltWattOperatingParametersPU/1 -> Bus Selector2/1

== system ESSLibrary/FilterResponse ==
  Enable : Inport
  SignalIn : Inport  Port=2
  LagTmConst : Inport  Port=3
  LeadTmConst : Inport  Port=4
  TimeStep : Inport  Port=5
  If : If  IfExpression=u1 ~= 0
  If Action Subsystem : Subsystem  TreatAsAtomicUnit=on
  If Action Subsystem1 : Subsystem  TreatAsAtomicUnit=on
  SignalIn1 : InportShadow  Port=2
  Switch1 : Switch  Criteria=u2 > Threshold
  Switch2 : Switch  Criteria=u2 > Threshold
  SignalOut : Outport  InitialOutput=0
  ErrorCode : Outport  Port=2  InitialOutput=0
  wires:
  Switch2/1 -> SignalOut/1
  Switch1/1 -> ErrorCode/1
  If/1 -> If Action Subsystem/Action
  If/2 -> If Action Subsystem1/Action
  LeadTmConst/1 -> If Action Subsystem/2(LeadTmConst)
  SignalIn/1 -> If Action Subsystem/1(SignalIn)
  SignalIn1/1 -> If Action Subsystem1/1(SignalIn)
  Enable/1 -> Switch2/2, Switch1/2, If/1
  TimeStep/1 -> If Action Subsystem/4(TimeStep)
  LagTmConst/1 -> If Action Subsystem/3(LagTmConst)
  If Action Subsystem1/2(ErrorCode) -> [ElseErrorCode]
  If Action Subsystem1/1(SignalOut) -> [ElseSignalOut]
  If Action Subsystem/2(ErrorCode) -> [IfErrorCode]
  If Action Subsystem/1(SignalOut) -> [IfSignalOut]
  [IfErrorCode] -> Switch1/1
  [ElseErrorCode] -> Switch1/3
  [ElseSignalOut] -> Switch2/3
  [IfSignalOut] -> Switch2/1

== system ESSLibrary/FixedPFMode ==
  PowerFactorSet : Inport
  ActivePowerMeasPU : Inport  Port=2
  LogicalBlockID : Inport  Port=3  OutDataTypeStr=int64
  Action Port : ActionPort
  Constant10 : Constant  Value=0  OutDataTypeStr=int64
  Constant11 : Constant  Value=0  OutDataTypeStr=int64
  Equal2 : RelationalOperator  Operator=>  OutDataTypeStr=boolean  RndMeth=Simplest
  Gain1 : Gain  Gain=1000000
  MATLAB Function : MATLAB Function  TreatAsAtomicUnit=on
  Sum2 : Sum  OutDataTypeStr=int64
  Switch4 : Switch  Criteria=u2 > Threshold
  ReactivePowerOut : Outport  OutDataTypeStr=double
  ErrorCode : Outport  Port=2  OutDataTypeStr=int64
  wires:
  PowerFactorSet/1 -> MATLAB Function/1(PowerFactorSet)
  ActivePowerMeasPU/1 -> MATLAB Function/2(ActivePowerMeasPU)
  MATLAB Function/1(ReactivePowerOut) -> ReactivePowerOut/1
  Constant10/1 -> Equal2/2
  Constant11/1 -> Switch4/3
  LogicalBlockID/1 -> Gain1/1
  Gain1/1 -> Sum2/2
  Equal2/1 -> Switch4/2
  Sum2/1 -> Switch4/1
  MATLAB Function/2(ErrorCode) -> Sum2/1, Equal2/1
  Switch4/1 -> ErrorCode/1

== system ESSLibrary/FrequencyWattMode ==
  FreqPU : Inport
  ActivePowerMeasPU : Inport  Port=2
  FreqWattOperatingParametersPU : Inport  Port=3  OutDataTypeStr=Bus: FreqWattOperatingParametersPU
  MaxDischargingPowerPU : Inport  Port=4  OutDataTypeStr=double
  MaxChargingPowerPU : Inport  Port=5  OutDataTypeStr=double
  LogicalBlockID : Inport  Port=6  OutDataTypeStr=int64
  Action Port : ActionPort
  Bus Selector4 : BusSelector  OutputSignals=FreqWattHiStartFreqPU,FreqWattHiStopFreqPU,FreqWattHiDischargeGradientPU,FreqWattHiChargeGradientPU,FreqWattLoStartFreqPU,FreqWattLoStopFreqPU,FreqWattLoDischargeGradientPU,FreqWattLoChargeGradientPU,FreqWattStartDelay,FreqWattStopDelay
  Comparator : $bdroot/ChargeDischargeStorageMode/Comparator  SystemSampleTime=-1  Latency=0  AutoFrameSizeCalculation=off
  Constant10 : Constant  Value=0  OutDataTypeStr=int64
  Constant11 : Constant  Value=0  OutDataTypeStr=int64
  Constant2 : Constant  Value=2  OutDataTypeStr=int32
  Constant3 : Constant  Value=0  OutDataTypeStr=int8
  Constant5 : Constant  Value=0  OutDataTypeStr=int8
  Constant6 : Constant  OutDataTypeStr=boolean
  Equal2 : RelationalOperator  Operator=>  OutDataTypeStr=boolean  RndMeth=Simplest
  Gain1 : Gain  Gain=1000000
  MATLAB Function : MATLAB Function  TreatAsAtomicUnit=on
  MaxChargingPowerPU1 : InportShadow  Port=5  OutDataTypeStr=double
  MaxDischargingPowerPU1 : InportShadow  Port=4  OutDataTypeStr=double
  SaturationLimits : $bdroot/SaturationLimits  SystemSampleTime=-1  Latency=0  AutoFrameSizeCalculation=off
  Sum2 : Sum  OutDataTypeStr=int64
  Switch4 : Switch  Criteria=u2 > Threshold
  Terminator : Terminator
  Terminator1 : Terminator
  VariableIdentifier : Constant  OutDataTypeStr=int64
  ActivePowerOut : Outport  OutDataTypeStr=double
  ErrorCode : Outport  Port=2  OutDataTypeStr=int64
  wires:
  Bus Selector4/7 -> [FreqWattLoDischargeGradientPU]  "<FreqWattLoDischargeGradientPU>"
  [FreqWattStopDelay] -> MATLAB Function/12(StopDelay)
  Bus Selector4/10 -> [FreqWattStopDelay]  "<FreqWattStopDelay>"
  Bus Selector4/4 -> [FreqWattHiChargeGradientPU]  "<FreqWattHiChargeGradientPU>"
  Bus Selector4/5 -> [FreqWattLoStartVoltagePU]  "<FreqWattLoStartFreqPU>"
  [FreqWattLoChargeGradientPU] -> MATLAB Function/10(LoX_NegativeY_Gradient)
  [FreqWattLoDischargeGradientPU] -> MATLAB Function/9(LoX_PositiveY_Gradient)
  [FreqWattLoStartVoltagePU] -> MATLAB Function/7(LoStartX)
  FreqPU/1 -> MATLAB Function/1(X_In)
  SaturationLimits/1 -> ActivePowerOut/1
  Constant10/1 -> Equal2/2
  MATLAB Function/1(Y_Out) -> SaturationLimits/1, Comparator/2
  Sum2/1 -> Switch4/1
  Comparator/3 -> Terminator1/1
  MaxDischargingPowerPU/1 -> SaturationLimits/2
  MaxChargingPowerPU1/1 -> Comparator/4
  MaxDischargingPowerPU1/1 -> Comparator/3
  Equal2/1 -> Switch4/2
  Bus Selector4/9 -> [FreqWattStartDelay]  "<FreqWattStartDelay>"
  Gain1/1 -> Sum2/2
  Constant11/1 -> Switch4/3
  Switch4/1 -> ErrorCode/1
  Comparator/2 -> Terminator/1
  Comparator/1 -> Equal2/1, Sum2/1
  Constant6/1 -> Comparator/1
  VariableIdentifier/1 -> Comparator/8
  Constant3/1 -> Comparator/6
  [FreqWattStartDelay] -> MATLAB Function/11(StartDelay)
  Constant2/1 -> Comparator/5
  Bus Selector4/3 -> [FreqWattHiDischargeGradientPU]  "<FreqWattHiDischargeGradientPU>"
  FreqWattOperatingParametersPU/1 -> Bus Selector4/1
  Constant5/1 -> Comparator/7
  Bus Selector4/2 -> [FreqWattHiStopVoltagePU]  "<FreqWattHiStopFreqPU>"
  [FreqWattHiChargeGradientPU] -> MATLAB Function/6(HiX_NegativeY_Gradient)
  LogicalBlockID/1 -> Gain1/1
  ActivePowerMeasPU/1 -> MATLAB Function/2(Y_In)
  [FreqWattLoStopVoltagePU] -> MATLAB Function/8(LoStopX)
  [FreqWattHiStopVoltagePU] -> MATLAB Function/4(HiStopX)
  [FreqWattHiDischargeGradientPU] -> MATLAB Function/5(HiX_PositiveY_Gradient)
  Bus Selector4/6 -> [FreqWattLoStopVoltagePU]  "<FreqWattLoStopFreqPU>"
  MaxChargingPowerPU/1 -> SaturationLimits/3
  Bus Selector4/8 -> [FreqWattLoChargeGradientPU]  "<FreqWattLoChargeGradientPU>"
  Bus Selector4/1 -> [FreqWattHiStartVoltagePU]  "<FreqWattHiStartFreqPU>"
  [FreqWattHiStartVoltagePU] -> MATLAB Function/3(HiStartX)

== system ESSLibrary/Manual ==
  Enable : Inport  OutDataTypeStr=boolean
  CommQual : Inport  Port=2  OutDataTypeStr=boolean
  OpenCmdIn : Inport  Port=3  OutDataTypeStr=boolean
  CloseCmdIn : Inport  Port=4  OutDataTypeStr=boolean
  FreqWithinLimits : Inport  Port=5  OutDataTypeStr=boolean
  VoltWithinLimits : Inport  Port=6  OutDataTypeStr=boolean
  ActivePowerSetPU : Inport  Port=7  OutDataTypeStr=double
  ReactivePowerSetPU : Inport  Port=8  OutDataTypeStr=double
  ZeroActivePowerFlow : Inport  Port=9  OutDataTypeStr=boolean
  ZeroReactivePowerFlow : Inport  Port=10  OutDataTypeStr=boolean
  CBStatus : Inport  Port=11  OutDataTypeStr=int8
  BreakerCmdTime : Inport  Port=12
  OpenTimeOut : Inport  Port=13
  CloseTimeOut : Inport  Port=14
  LogicalBlockID : Inport  Port=15  OutDataTypeStr=int64
  AND : Logic  IconShape=distinctive  AllPortsSameDT=off  OutDataTypeStr=boolean
  ElseActionSubsystem : Subsystem  TreatAsAtomicUnit=on
  If : If  IfExpression=u1 ~= 0
  IfActionSubsystem : Subsystem  TreatAsAtomicUnit=on
  NOT : Logic  Operator=NOT  IconShape=distinctive  AllPortsSameDT=off  OutDataTypeStr=boolean
  Switch{,1..4} (5 alike) : Switch  Criteria=u2 > Threshold
  ActivePowerOut : Outport
  ReactivePowerOut : Outport  Port=2
  OpenCmd : Outport  Port=3
  CloseCmd : Outport  Port=4
  ErrorCode : Outport  Port=5  OutDataTypeStr=int64
  wires:
  NOT/1 -> AND/2
  Enable/1 -> AND/1
  CommQual/1 -> NOT/1
  If/1 -> IfActionSubsystem/Action
  If/2 -> ElseActionSubsystem/Action
  ElseActionSubsystem/1(ActivePowerOut) -> [ElseActivePowerOut]
  ElseActionSubsystem/5(ErrorCode) -> [ElseErrorCode]
  ElseActionSubsystem/3(OpenCmd) -> [ElseOpenCmd]
  ElseActionSubsystem/4(CloseCmd) -> [ElseCloseCmd]
  ElseActionSubsystem/2(ReactivePowerOut) -> [ElseReactivePowerOut]
  IfActionSubsystem/5(ErrorCode) -> [IfErrorCode]
  IfActionSubsystem/4(CloseCmd) -> [IfCloseCmd]
  IfActionSubsystem/3(OpenCmd) -> [IfOpenCmd]
  IfActionSubsystem/2(ReactivePowerOut) -> [IfReactivePowerOut]
  IfActionSubsystem/1(ActivePowerOut) -> [IfActivePowerOut]
  OpenCmdIn/1 -> IfActionSubsystem/1(OpenCmdIn)
  CloseCmdIn/1 -> IfActionSubsystem/2(CloseCmdIn)
  FreqWithinLimits/1 -> IfActionSubsystem/3(FreqWithinLimits)
  VoltWithinLimits/1 -> IfActionSubsystem/4(VoltWithinLimits)
  ActivePowerSetPU/1 -> IfActionSubsystem/5(ActivePowerSetPU)
  ReactivePowerSetPU/1 -> IfActionSubsystem/6(ReactivePowerSetPU)
  ZeroActivePowerFlow/1 -> IfActionSubsystem/7(ZeroActivePowerFlow)
  ZeroReactivePowerFlow/1 -> IfActionSubsystem/8(ZeroReactivePowerFlow)
  CBStatus/1 -> IfActionSubsystem/9(CBStatus)
  BreakerCmdTime/1 -> IfActionSubsystem/10(BreakerCmdTime)
  LogicalBlockID/1 -> IfActionSubsystem/13(LogicalBlockID)
  [ElseErrorCode] -> Switch4/3
  AND/1 -> Switch4/2, Switch3/2, Switch2/2, Switch1/2, Switch/2, If/1
  Switch1/1 -> ReactivePowerOut/1
  Switch4/1 -> ErrorCode/1
  [IfActivePowerOut] -> Switch/1
  [IfErrorCode] -> Switch4/1
  [IfOpenCmd] -> Switch2/1
  [ElseOpenCmd] -> Switch2/3
  Switch2/1 -> OpenCmd/1
  [IfCloseCmd] -> Switch3/1
  [IfReactivePowerOut] -> Switch1/1
  [ElseReactivePowerOut] -> Switch1/3
  [ElseCloseCmd] -> Switch3/3
  [ElseActivePowerOut] -> Switch/3
  Switch/1 -> ActivePowerOut/1
  Switch3/1 -> CloseCmd/1
  OpenTimeOut/1 -> IfActionSubsystem/11(OpenTimeOut)
  CloseTimeOut/1 -> IfActionSubsystem/12(CloseTimeOut)

== system ESSLibrary/MovAvgDeltaVoltCalc1 ==
  Enable : Inport
  Inp : Inport  Port=2
  FilterTime : Inport  Port=3
  TimeStep : Inport  Port=4
  ElseMovAvgFilter : Subsystem  TreatAsAtomicUnit=on
  If : If  IfExpression=u1 ~= 0
  IfMovAvgFilter : Subsystem  TreatAsAtomicUnit=on
  Inp1 : InportShadow  Port=2
  Switch : Switch  Criteria=u2 > Threshold
  Switch1 : Switch  Criteria=u2 > Threshold
  Out : Outport
  ErrorCode : Outport  Port=2
  wires:
  [ElseErrorCode] -> Switch1/3
  [IfErrorCode] -> Switch1/1
  [IfOut] -> Switch/1
  [ElseOut] -> Switch/3
  Switch/1 -> Out/1
  Switch1/1 -> ErrorCode/1
  IfMovAvgFilter/2(ErrorCode) -> [IfErrorCode]
  IfMovAvgFilter/1(Out) -> [IfOut]
  ElseMovAvgFilter/2(ErrorCode) -> [ElseErrorCode]
  ElseMovAvgFilter/1(Out) -> [ElseOut]
  Inp1/1 -> ElseMovAvgFilter/1(Inp)
  FilterTime/1 -> IfMovAvgFilter/2(FilterTime)
  TimeStep/1 -> IfMovAvgFilter/3(TimeStep)
  Inp/1 -> IfMovAvgFilter/1(Inp)
  If/1 -> IfMovAvgFilter/Action
  If/2 -> ElseMovAvgFilter/Action
  Enable/1 -> If/1, Switch/2, Switch1/2

== system ESSLibrary/OperationModeSelector ==
  Enable : Inport  OutDataTypeStr=boolean
  OperationMode : Inport  Port=2  OutDataTypeStr=int8
  LogicalBlockID : Inport  Port=3  OutDataTypeStr=int64
  ElseActionSubsystem : Subsystem  TreatAsAtomicUnit=on
  If : If  IfExpression=u1 ~= 0
  IfAction Subsystem : Subsystem  TreatAsAtomicUnit=on
  Switch : Switch  Criteria=u2 > Threshold
  Switch1 : Switch  Criteria=u2 > Threshold
  Switch2 : Switch  Criteria=u2 > Threshold
  Switch3 : Switch  Criteria=u2 > Threshold  OutDataTypeStr=int64
  EnableDisconnected : Outport
  EnableManual : Outport  Port=2
  EnableAuto : Outport  Port=3
  ErrorCode : Outport  Port=4  OutDataTypeStr=int64
  wires:
  Enable/1 -> Switch/2, Switch1/2, Switch2/2, Switch3/2, If/1
  If/1 -> IfAction Subsystem/Action
  OperationMode/1 -> IfAction Subsystem/1(OperationMode)
  IfAction Subsystem/1(EnableDisconnected) -> [EnableDisconnectedIf]
  IfAction Subsystem/2(EnableManual) -> [EnableManualIf]
  IfAction Subsystem/3(EnableAuto) -> [EnableAutoIf]
  Switch/1 -> EnableDisconnected/1
  Switch1/1 -> EnableManual/1
  Switch2/1 -> EnableAuto/1
  [EnableDisconnectedIf] -> Switch/1
  [EnableDisconnectedElse] -> Switch/3
  [EnableManualIf] -> Switch1/1
  [EnableManualElse] -> Switch1/3
  [EnableAutoIf] -> Switch2/1
  [EnableAutoElse] -> Switch2/3
  [EnableErrCdElse] -> Switch3/3
  [EnableErrCdIf] -> Switch3/1
  IfAction Subsystem/4(ErrorCodeOut) -> [EnableErrCdIf]
  Switch3/1 -> ErrorCode/1
  If/2 -> ElseActionSubsystem/Action
  LogicalBlockID/1 -> IfAction Subsystem/2(LogicalBlockID)
  ElseActionSubsystem/1(EnableDisconnected) -> [EnableDisconnectedElse]
  ElseActionSubsystem/2(EnableManual) -> [EnableManualElse]
  ElseActionSubsystem/3(EnableAuto) -> [EnableAutoElse]
  ElseActionSubsystem/4(ErrorCodeOut) -> [EnableErrCdElse]

== system ESSLibrary/PFReference_P ==
  EnableDisable : Inport
  PFLimit : Inport  Port=2
  PValPFLimit : Inport  Port=3
  PValPF1 : Inport  Port=4
  PSet : Inport  Port=5
  Enable1 : InportShadow
  If : If  IfExpression=u1 ~= 0
  If Action Subsystem : Subsystem  TreatAsAtomicUnit=on
  If Action Subsystem1 : Subsystem  TreatAsAtomicUnit=on
  Switch : Switch  Criteria=u2 > Threshold
  Switch2 : Switch  Criteria=u2 > Threshold
  PFSet : Outport
  ErrorCode : Outport  Port=2
  wires:
  [IfErrorCode] -> Switch/1
  [ElseErrorCode] -> Switch/3
  If Action Subsystem/2(ErrorCode) -> [IfErrorCode]
  If Action Subsystem1/2(ErrorCode) -> [ElseErrorCode]
  Enable1/1 -> Switch/2, Switch2/2
  Switch/1 -> ErrorCode/1
  PSet/1 -> If Action Subsystem/4(PSet)
  PValPF1/1 -> If Action Subsystem/3(PValPF1)
  PValPFLimit/1 -> If Action Subsystem/2(PValPFLimit)
  PFLimit/1 -> If Action Subsystem/1(PFLimit)
  If/2 -> If Action Subsystem1/Action
  If/1 -> If Action Subsystem/Action
  EnableDisable/1 -> If/1
  If Action Subsystem1/1(ElsePFSet) -> [ElsePFSet]
  [PFSet] -> Switch2/1
  [ElsePFSet] -> Switch2/3
  Switch2/1 -> PFSet/1
  If Action Subsystem/1(PFSet) -> [PFSet]

== system ESSLibrary/PIController ==
  Enable : Inport
  ErrSig : Inport  Port=2
  Kp : Inport  Port=3
  Ki : Inport  Port=4
  TimeStep : Inport  Port=5
  HighLimit : Inport  Port=6
  LowLimit : Inport  Port=7
  Enable1 : InportShadow
  If : If  IfExpression=u1 ~= 0
  If Action Subsystem : Subsystem  TreatAsAtomicUnit=on
  If Action Subsystem1 : Subsystem  TreatAsAtomicUnit=on
  Switch : Switch  Criteria=u2 > Threshold
  Switch1 : Switch  Criteria=u2 > Threshold
  CtrlSig : Outport  InitialOutput=0
  ErrorCode : Outport  Port=2  InitialOutput=0
  wires:
  Enable/1 -> If/1
  If/2 -> If Action Subsystem1/Action
  If/1 -> If Action Subsystem/Action
  ErrSig/1 -> If Action Subsystem/1(ErrSig)
  Kp/1 -> If Action Subsystem/2(Kp)
  Ki/1 -> If Action Subsystem/3(Ki)
  TimeStep/1 -> If Action Subsystem/4(TimeStep)
  HighLimit/1 -> If Action Subsystem/5(HighLimit)
  LowLimit/1 -> If Action Subsystem/6(LowLimit)
  If Action Subsystem/1(CntrSig) -> [IfOut]
  [IfOut] -> Switch/1
  [ElseOut] -> Switch/3
  Switch/1 -> CtrlSig/1
  If Action Subsystem1/1(Out) -> [ElseOut]
  [IfErrorCode] -> Switch1/1
  [ElseErrorCode] -> Switch1/3
  Switch1/1 -> ErrorCode/1
  Enable1/1 -> Switch1/2, Switch/2
  If Action Subsystem1/2(ErrorCode) -> [ElseErrorCode]
  If Action Subsystem/2(ErrorCode) -> [IfErrorCode]
